simulink model "model"  (R2020b)
settings: Solver=VariableStepAuto  StartTime=0.0  StopTime=settings.Tsim  FixedStep=0.1  RelTol=1e-6  AbsTol=1e-6
values from neighbouring files (symbols this model uses):
  D = date(3)    [date2jd.m]
  settings = Simulink.Parameter    [main.m]
libraries: vrlib x10
(part 1 of 2)
settings Model: Creator=rosat  LastModifiedBy=rosat
settings SolverCC: ZeroCrossAlgorithm=Adaptive
settings OptimizationCC: BlockReduction=off  DefaultParameterBehavior=Inlined  BufferReuse=off
settings DebuggingCC: IgnoredZcDiagnostic=none  SFMachineParentedDataDiag=error

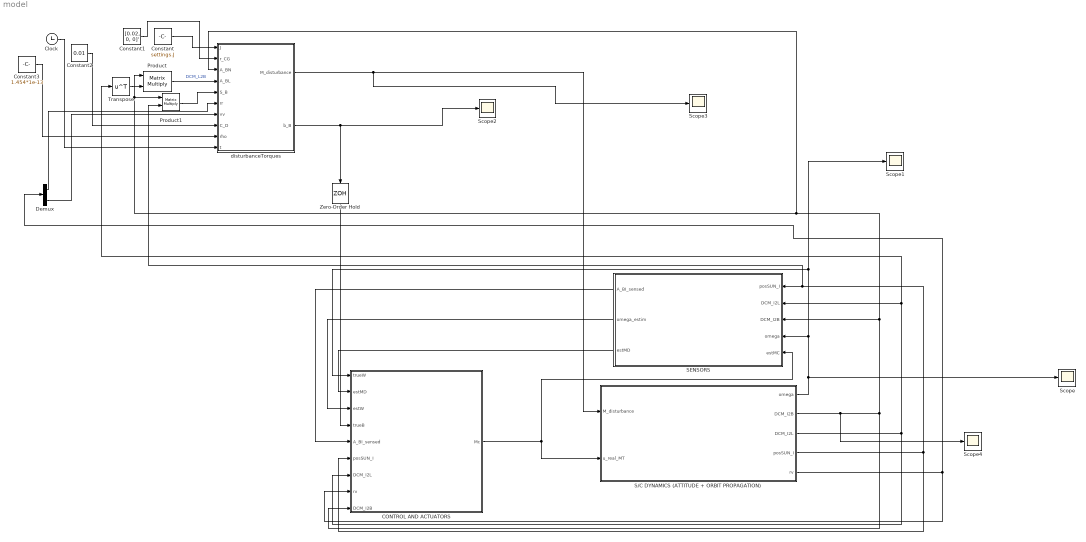
== system model ==
  CONTROL AND ACTUATORS : Subsystem
  Clock : Clock
  Constant : Constant  Value=settings.J
  Constant1 : Constant  Value=[0.02, 0, 0]'
  Constant2 : Constant  Value=0.01
  Constant3 : Constant  Value=1.454*1e-13
  Demux : Demux  Outputs=2
  Product : Product  Multiplication=Matrix(*)
  Product1 : Product  Multiplication=Matrix(*)
  S/C DYNAMICS (ATTITUDE + ORBIT PROPAGATION) : Subsystem
  SENSORS : Subsystem
  Scope{,1..4} (5 alike) : Scope
  Transpose : Math  Operator=transpose  SaturateOnIntegerOverflow=on
  Zero-Order Hold : ZeroOrderHold  SampleTime=0.01
  disturbanceTorques : MATLAB Function  TreatAsAtomicUnit=on
  wires:
  Constant/1 -> disturbanceTorques/1(J)
  Constant1/1 -> disturbanceTorques/2(r_CG)
  Transpose/1 -> Product/2
  Product/1 -> disturbanceTorques/4(A_BL)  "DCM_L2B"
  Product1/1 -> disturbanceTorques/5(S_B)
  Demux/1 -> disturbanceTorques/6(rr)
  Demux/2 -> disturbanceTorques/7(vv)
  Constant2/1 -> disturbanceTorques/8(C_D)
  Constant3/1 -> disturbanceTorques/9(rho)
  Clock/1 -> disturbanceTorques/10(t)
  disturbanceTorques/1(M_disturbance) -> Scope3/1, S/C DYNAMICS (ATTITUDE + ORBIT PROPAGATION)/1(M_disturbance)
  disturbanceTorques/2(b_B) -> Scope2/1, Zero-Order Hold/1
  Zero-Order Hold/1 -> CONTROL AND ACTUATORS/4(trueB)
  S/C DYNAMICS (ATTITUDE + ORBIT PROPAGATION)/3(DCM_I2L) -> Transpose/1, SENSORS/2(DCM_I2L), CONTROL AND ACTUATORS/7(DCM_I2L)
  S/C DYNAMICS (ATTITUDE + ORBIT PROPAGATION)/4(posSUN_I) -> Product1/2, SENSORS/1(posSUN_I), CONTROL AND ACTUATORS/6(posSUN_I)
  S/C DYNAMICS (ATTITUDE + ORBIT PROPAGATION)/1(omega) -> Scope1/1, CONTROL AND ACTUATORS/1(trueW), SENSORS/4(omega), Scope/1
  S/C DYNAMICS (ATTITUDE + ORBIT PROPAGATION)/2(DCM_I2B) -> Scope4/1, disturbanceTorques/3(A_BN), Product1/1, Product/1, SENSORS/3(DCM_I2B), CONTROL AND ACTUATORS/9(DCM_I2B)
  S/C DYNAMICS (ATTITUDE + ORBIT PROPAGATION)/5(rv) -> Demux/1, CONTROL AND ACTUATORS/8(rv)
  SENSORS/2(omega_estim) -> CONTROL AND ACTUATORS/3(estW)
  SENSORS/3(estMD) -> CONTROL AND ACTUATORS/2(estMD)
  SENSORS/1(A_BI_sensed) -> CONTROL AND ACTUATORS/5(A_BI_sensed)
  CONTROL AND ACTUATORS/1(Mc) -> S/C DYNAMICS (ATTITUDE + ORBIT PROPAGATION)/2(u_real_MT), SENSORS/5(estMC)

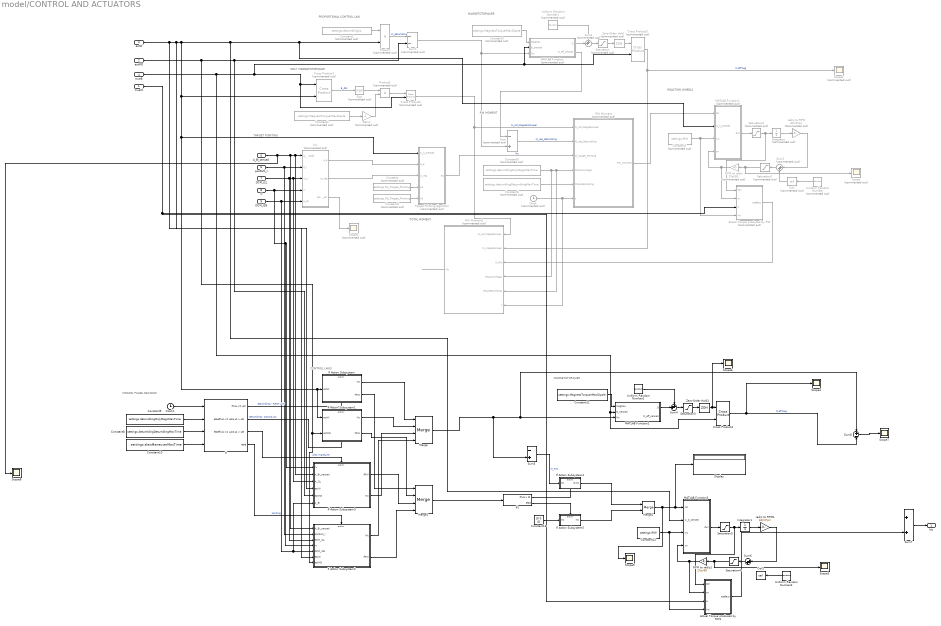
== system model/CONTROL AND ACTUATORS ==
  note: CONTROL LAWS
  note: MISSION PHASE DECISION
  note: TOTAL MOMENT
  note: REACTION WHEELS
  note: RW MOMENT
  note: TARGET POINTING
  note: MAGNETOTORQUER
  note: ONLY MAGNETOTORQUER
  note: PROPORTIONAL CONTROL LAW
  note: MAGNETOTORQUER
  trueW : Inport
  estMD : Inport  Port=2
  estW : Inport  Port=3
  trueB : Inport  Port=4
  A_BI_sensed : Inport  Port=5
  posSUN_I : Inport  Port=6
  DCM_I2L : Inport  Port=7
  rv : Inport  Port=8
  DCM_I2B : Inport  Port=9
  Actual Torque produced by RW : MATLAB Function  Commented=on  TreatAsAtomicUnit=on
  Actual Torque produced by RW1 : MATLAB Function  TreatAsAtomicUnit=on
  Ceil : Rounding  Commented=on  Operator=ceil
  Ceil1 : Rounding  Operator=ceil
  Clock : Clock  Commented=on
  Clock1 : Clock
  Constant : Constant  Commented=on  Value=settings.Kp_Target_Pointing
  Constant1 : Constant  Commented=on  Value=settings.detumblingkp
  Constant10 : Constant  Value=settings.slewManeuverMaxTime
  Constant11 : Constant  Value=settings.MagnetoTorquerMaxDipole
  Constant12 : Constant  Value=settings.IRW
  Constant13 : Constant  Value=[0 0 0]
  Constant2 : Constant  Commented=on  Value=settings.MagnetoTorquerMaxDipole
  Constant3 : Constant  Commented=on  Value=settings.MagnetoTorquerMaxDipole
  Constant4 : Constant  Commented=on  Value=settings.Kd_Target_Pointing
  Constant5 : Constant  Commented=on  Value=settings.detumblingOnlyMagnMaxTime
  Constant6 : Constant  Commented=on  Value=settings.detumblingDetumblingMaxTime
  Constant7 : Constant  Commented=on  Value=settings.IRW
  Constant8 : Constant  Value=settings.detumblingDetumblingMaxTime
  Constant9 : Constant  Value=settings.detumblingOnlyMagnMaxTime
  Cross Product1 : vrlib/Utilities/Cross Product  Commented=on
  Cross Product2 : vrlib/Utilities/Cross Product  Commented=on
  Cross Product3 : vrlib/Utilities/Cross Product  Commented=on
  Cross Product4 : vrlib/Utilities/Cross Product
  Display : Display
  Gain1 : Gain  Commented=on  Gain=-1
  If : If  NumInputs=4  IfExpression=u1 <= u2  ElseIfExpressions=u1 <= u3 & u1 > u2, u1 <= u4 & u1 > u3
  If Action Subsystem : Subsystem  TreatAsAtomicUnit=on
  If Action Subsystem1 : Subsystem  TreatAsAtomicUnit=on
  If Action Subsystem2 : Subsystem  TreatAsAtomicUnit=on
  If Action Subsystem3 : Subsystem  TreatAsAtomicUnit=on
  If Action Subsystem4 : Subsystem  TreatAsAtomicUnit=on
  If Action Subsystem5 : Subsystem  TreatAsAtomicUnit=on
  If1 : If
  Integrator : Integrator  Commented=on  InitialCondition=[0;0;0]
  Integrator1 : Integrator  InitialCondition=[0;0;0]
  MATLAB Function : MATLAB Function  Commented=on  TreatAsAtomicUnit=on
  MATLAB Function1 : MATLAB Function  Commented=on  TreatAsAtomicUnit=on
  MATLAB Function2 : MATLAB Function  TreatAsAtomicUnit=on
  MATLAB Function3 : MATLAB Function  TreatAsAtomicUnit=on
  Merge : Merge  Inputs=4
  Merge1 : Merge  Inputs=4
  Merge2 : Merge
  Product : Product  Commented=on
  Product1 : Product  Commented=on
  RPM to rad/s : Gain  Commented=on  Gain=2*pi/60
  RPM to rad/s1 : Gain  Gain=2*pi/60
  RW Moment : MATLAB Function  Commented=on  TreatAsAtomicUnit=on
  RW Moment1 : MATLAB Function  Commented=on  TreatAsAtomicUnit=on
  Saturation : Saturate  Commented=on  UpperLimit=settings.MagnetoTorquerMaxDipole  LowerLimit=-settings.MagnetoTorquerMaxDipole
  Saturation1 : Saturate  Commented=on  UpperLimit=settings.MaxRPM*[1;1;1]  LowerLimit=-settings.MaxRPM*[1;1;1]  LinearizeAsGain=off  ZeroCross=off
  Saturation2 : Saturate  Commented=on  UpperLimit=settings.MaxRPM_Rate  LowerLimit=-settings.MaxRPM_Rate
  Saturation3 : Saturate  UpperLimit=settings.MagnetoTorquerMaxDipole  LowerLimit=-settings.MagnetoTorquerMaxDipole
  Saturation4 : Saturate  UpperLimit=settings.MaxRPM*[1;1;1]  LowerLimit=-settings.MaxRPM*[1;1;1]  LinearizeAsGain=off  ZeroCross=off
  Saturation5 : Saturate  UpperLimit=settings.MaxRPM_Rate  LowerLimit=-settings.MaxRPM_Rate
  Scope : Scope  Commented=on
  Scope1 : Scope  Commented=on
  Scope2 : Scope  Commented=on
  Scope{3..8} (6 alike) : Scope
  Sign : Signum  Commented=on
  Sum : Sum  Commented=on  Inputs=-+
  Sum1 : Sum  Commented=on  Inputs=--
  Sum2 : Sum  Commented=on  Inputs=++|
  Sum3 : Sum  Commented=on  Inputs=|++
  Sum4 : Sum  Inputs=++|
  Sum5 : Sum  Inputs=-+
  Sum6 : Sum  Inputs=|++
  Sum7 : Sum
  Sum8 : Sum  Inputs=+-
  Target Pointing Algorithm : MATLAB Function  Commented=on  TreatAsAtomicUnit=on
  Uniform Random Number : UniformRandomNumber  Commented=on  Minimum=-settings.RPMAccuracy*[1;1;1]  Maximum=settings.RPMAccuracy*[1;1;1]  Seed=561651  SampleTime=1/settings.RW_sr
  Uniform Random Number1 : UniformRandomNumber  Commented=on  Minimum=-settings.MagnetoTorquerDipoleError*[1;1;1]  Maximum=settings.MagnetoTorquerDipoleError*[1;1;1]  Seed=456156  SampleTime=1/settings.MagnetoTorquerSampleRate
  Uniform Random Number2 : UniformRandomNumber  Minimum=-settings.MagnetoTorquerDipoleError*[1;1;1]  Maximum=settings.MagnetoTorquerDipoleError*[1;1;1]  Seed=456156  SampleTime=1/settings.MagnetoTorquerSampleRate
  Uniform Random Number3 : UniformRandomNumber  Minimum=-settings.RPMAccuracy*[1;1;1]  Maximum=settings.RPMAccuracy*[1;1;1]  Seed=561651  SampleTime=1/settings.RW_sr
  Zero-Order Hold : ZeroOrderHold  Commented=on  SampleTime=1/settings.MagnetoTorquerSampleRate
  Zero-Order Hold1 : ZeroOrderHold  SampleTime=1/settings.MagnetoTorquerSampleRate
  fcn : MATLAB Function  Commented=on  TreatAsAtomicUnit=on
  rad/s to RPM : Gain  Commented=on  Gain=60/(2*pi)
  rad/s to RPM1 : Gain  Gain=60/(2*pi)
  Mc : Outport
  wires:
  Constant1/1 -> Product/1
  Cross Product2/1 -> RW Moment1/1(M_onlyMagnetorquer), RW Moment/1(M_onlyMagnetorquer)  "M_onlyMagnetotorquer"
  Constant2/1 -> Gain1/1
  Cross Product1/1 -> Sign/1  "B_dot"
  Gain1/1 -> Product1/2
  Sign/1 -> Product1/1
  Product1/1 -> Cross Product2/1
  MATLAB Function/2(M_eff_sensed) -> Sum/1
  Uniform Random Number1/1 -> Sum2/1
  Zero-Order Hold/1 -> Cross Product3/1
  MATLAB Function/1(D) -> Sum2/2
  Sum2/1 -> Saturation/1
  Saturation/1 -> Zero-Order Hold/1
  Cross Product3/1 -> Scope1/1, RW Moment1/2(M_magnetorquer)  "M eff Mag"
  Constant3/1 -> MATLAB Function/1(MagMax)
  Sum/1 -> RW Moment/2(M_req_Detumbling)  "M_req_detumbling"
  Product/1 -> Sum1/1  "M_detumbling"
  Sum1/1 -> Sum/2, MATLAB Function/3(Mc)
  fcn/1(A_e) -> Target Pointing Algorithm/2(A_e)
  DCM_I2L/1 -> If Action Subsystem2/3(DCM_I2L), If Action Subsystem3/3(A_I2L), fcn/3(A_LI)
  Target Pointing Algorithm/1(Mc) -> RW Moment/3(M_Target_Pointing)  "Mc"
  A_BI_sensed/1 -> Scope8/1, If Action Subsystem3/2(A_BI_sensed), fcn/1(A_BI_sensed), If Action Subsystem2/1(A_BI_sensed)
  Constant/1 -> Target Pointing Algorithm/4(Kp)
  Constant4/1 -> Target Pointing Algorithm/5(Kd)
  posSUN_I/1 -> If Action Subsystem2/2(posSUN_I), fcn/2(S_I)
  DCM_I2B/1 -> If Action Subsystem3/6(A_BI), If Action Subsystem2/5(DCM_I2B), fcn/5(A_BI)
  fcn/3(pointing_err) -> Scope2/1
  rv/1 -> If Action Subsystem3/1(rv), If Action Subsystem2/4(rv), fcn/4(rv)
  fcn/2(w_req) -> Target Pointing Algorithm/3(w_req)
  Constant5/1 -> RW Moment1/4(tMaxOnlyMagn), RW Moment1/5(tMaxDetumbling), RW Moment/4(tMaxOnlyMagn)
  Constant6/1 -> RW Moment/5(tMaxDetumbling)
  Clock/1 -> RW Moment1/6(t), RW Moment/6(t)
  RW Moment/1(RW_Moment) -> MATLAB Function1/1(Mc)
  Actual Torque produced by RW/1(MeffRW) -> RW Moment1/3(M_RW)
  Ceil/1 -> Sum3/2
  Sum3/1 -> Saturation1/1
  Saturation1/1 -> Scope/1, RPM to rad/s/1
  Integrator/1 -> rad/s to RPM/1
  MATLAB Function1/1(dwr) -> Saturation2/1
  Constant7/1 -> Actual Torque produced by RW/4(Irw), MATLAB Function1/3(Irw)
  RPM to rad/s/1 -> Actual Torque produced by RW/2(wr), MATLAB Function1/4(wr)
  trueW/1 -> Actual Torque produced by RW1/3(w), Actual Torque produced by RW/3(w)
  Uniform Random Number/1 -> Ceil/1
  rad/s to RPM/1 -> Sum3/1
  Saturation2/1 -> Actual Torque produced by RW/1(dwr), Integrator/1
  RW Moment1/1(Mc) -> ?
  Clock1/1 -> If/1
  Constant9/1 -> If/2
  Constant8/1 -> If/3
  If/1 -> If Action Subsystem/Action  "detumbling - FIRST LAW"
  If/2 -> If Action Subsystem1/Action  "detumbling - second law"
  If/4 -> If Action Subsystem2/Action  "pointing"
  Constant10/1 -> If/4
  If/3 -> If Action Subsystem3/Action  "slew maneuver"
  estW/1 -> If Action Subsystem2/6(estW), If Action Subsystem3/4(estW), If Action Subsystem1/1(estW), If Action Subsystem/1(estW), Target Pointing Algorithm/1(w_b_sensed), Cross Product1/2, MATLAB Function3/2(w_b_sensed), MATLAB Function1/2(w_b_sensed), Product/2
  trueB/1 -> Cross Product4/2, MATLAB Function2/2(B_sensed), Cross Product3/2, MATLAB Function/2(B_sensed), Cross Product2/2, Cross Product1/1
  Sum4/1 -> Saturation3/1
  Zero-Order Hold1/1 -> Scope6/1, Cross Product4/1
  Constant11/1 -> MATLAB Function2/1(MagMax)
  MATLAB Function2/1(D) -> Sum4/2
  Saturation3/1 -> Zero-Order Hold1/1
  Uniform Random Number2/1 -> Sum4/1
  If Action Subsystem/1(Mc) -> Merge/1
  If Action Subsystem1/1(Mc) -> Merge/2
  If Action Subsystem/2(ifRW) -> Merge1/1
  If Action Subsystem1/2(ifRW) -> Merge1/2
  If Action Subsystem2/2(ifRW) -> Merge1/4
  If Action Subsystem2/1(Mc) -> Merge/4
  If Action Subsystem3/2(Mc) -> Merge/3
  If Action Subsystem3/1(ifRW) -> Merge1/3
  Merge/1 -> Sum5/2, Sum8/1, MATLAB Function2/3(Mc)
  estMD/1 -> If Action Subsystem2/7(estMD), If Action Subsystem1/2(estMD), If Action Subsystem3/5(estMD), Sum1/2
  Merge1/1 -> If1/1
  Cross Product4/1 -> Scope4/1, Sum8/2  "M eff Mag"
  Sum5/1 -> If Action Subsystem4/1(In1)  "M_RW"
  rad/s to RPM1/1 -> Sum6/1
  Uniform Random Number3/1 -> Ceil1/1
  RPM to rad/s1/1 -> Actual Torque produced by RW1/2(wr), MATLAB Function3/4(wr)
  Constant12/1 -> Actual Torque produced by RW1/4(Irw), MATLAB Function3/3(Irw)
  MATLAB Function3/1(dwr) -> Saturation5/1
  Saturation4/1 -> Scope3/1, RPM to rad/s1/1
  Sum6/1 -> Saturation4/1
  Integrator1/1 -> rad/s to RPM1/1
  Saturation5/1 -> Actual Torque produced by RW1/1(dwr), Integrator1/1
  If1/1 -> If Action Subsystem4/Action
  If1/2 -> If Action Subsystem5/Action
  Constant13/1 -> If Action Subsystem5/1(In1)
  Merge2/1 -> Scope5/1, Display/1, MATLAB Function3/1(Mc)
  If Action Subsystem4/1(Out1) -> Merge2/1
  If Action Subsystem5/1(Mc) -> Merge2/2
  Sum7/1 -> Mc/1
  Sum8/1 -> Scope7/1
  Actual Torque produced by RW1/1(MeffRW) -> Sum7/2

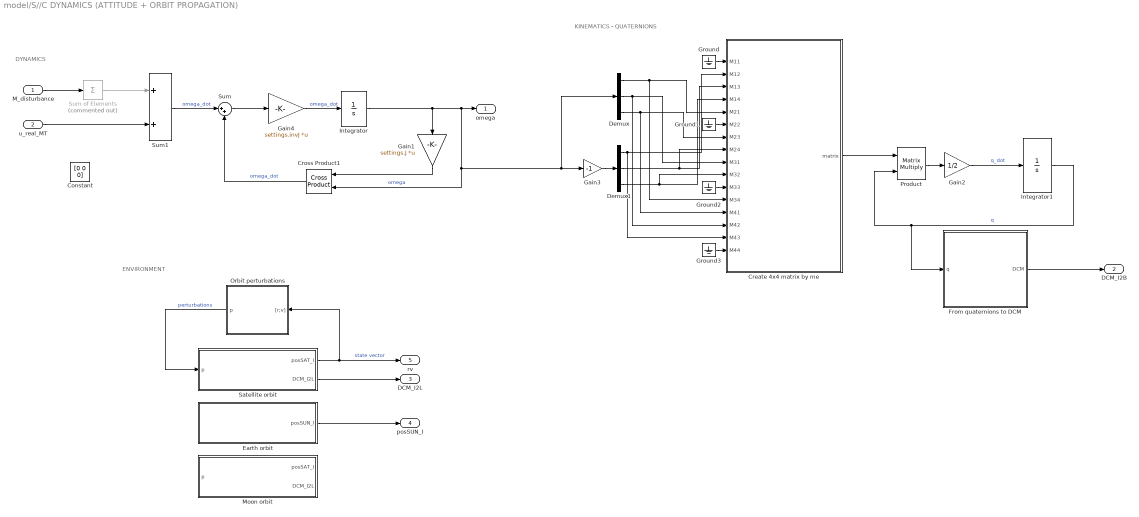
== system model/S//C DYNAMICS (ATTITUDE + ORBIT PROPAGATION) ==
  note: ENVIRONMENT
  note: KINEMATICS - QUATERNIONS
  note: DYNAMICS
  M_disturbance : Inport
  u_real_MT : Inport  Port=2
  Constant : Constant  Value=[0 0 0]
  Create 4x4 matrix by me : Subsystem
  Cross Product1 : vrlib/Utilities/Cross Product
  Demux : Demux  Outputs=3
  Demux1 : Demux  Outputs=3
  Earth orbit : Subsystem
  From quaternions to DCM : Subsystem
  Gain1 : Gain  Gain=settings.J  Multiplication=Matrix(K*u)
  Gain2 : Gain  Gain=1/2
  Gain3 : Gain  Gain=-1
  Gain4 : Gain  Gain=settings.invJ  Multiplication=Matrix(K*u)
  Ground{,1..3} (4 alike) : Ground
  Integrator : Integrator  InitialCondition=settings.omega0
  Integrator1 : Integrator  InitialCondition=settings.q0
  Moon orbit : Subsystem
  Orbit perturbations : Subsystem
  Product : Product  Multiplication=Matrix(*)
  Satellite orbit : Subsystem
  Sum : Sum  Inputs=|++
  Sum of Elements : Sum  Commented=on  Inputs=+  CollapseMode=Specified dimension  CollapseDim=2
  Sum1 : Sum
  omega : Outport
  DCM_I2B : Outport  Port=2
  DCM_I2L : Outport  Port=3
  posSUN_I : Outport  Port=4
  rv : Outport  Port=5
  wires:
  Sum of Elements/1 -> Sum1/1
  Integrator/1 -> Gain1/1, Demux/1, Gain3/1, Cross Product1/2, omega/1  "omega"
  Sum/1 -> Gain4/1
  u_real_MT/1 -> Sum1/2
  Sum1/1 -> Sum/1  "omega_dot"
  Gain4/1 -> Integrator/1  "omega_dot"
  Cross Product1/1 -> Sum/2  "omega_dot"
  Gain1/1 -> Cross Product1/1
  M_disturbance/1 -> Sum of Elements/1
  Demux/3 -> Create 4x4 matrix by me/13(M41), Create 4x4 matrix by me/7(M23)
  Product/1 -> Gain2/1
  Demux1/2 -> Create 4x4 matrix by me/8(M24), Create 4x4 matrix by me/3(M13)
  Demux1/3 -> Create 4x4 matrix by me/10(M32), Create 4x4 matrix by me/4(M14)
  Demux1/1 -> Create 4x4 matrix by me/15(M43), Create 4x4 matrix by me/2(M12)
  Demux/1 -> Create 4x4 matrix by me/12(M34), Create 4x4 matrix by me/5(M21)
  Ground2/1 -> Create 4x4 matrix by me/11(M33)
  Ground/1 -> Create 4x4 matrix by me/1(M11)
  From quaternions to DCM/1(DCM) -> DCM_I2B/1
  Demux/2 -> Create 4x4 matrix by me/14(M42), Create 4x4 matrix by me/9(M31)
  Ground3/1 -> Create 4x4 matrix by me/16(M44)
  Gain2/1 -> Integrator1/1  "q_dot"
  Integrator1/1 -> From quaternions to DCM/1(q), Product/2  "q"
  Gain3/1 -> Demux1/1
  Ground1/1 -> Create 4x4 matrix by me/6(M22)
  Create 4x4 matrix by me/1(matrix) -> Product/1
  Earth orbit/1(posSUN_I) -> posSUN_I/1
  Satellite orbit/1(posSAT_I) -> Orbit perturbations/1("[r;v]"), rv/1  "state vector"
  Orbit perturbations/1(p) -> Satellite orbit/1(p)  "perturbations"
  Satellite orbit/2(DCM_I2L) -> DCM_I2L/1

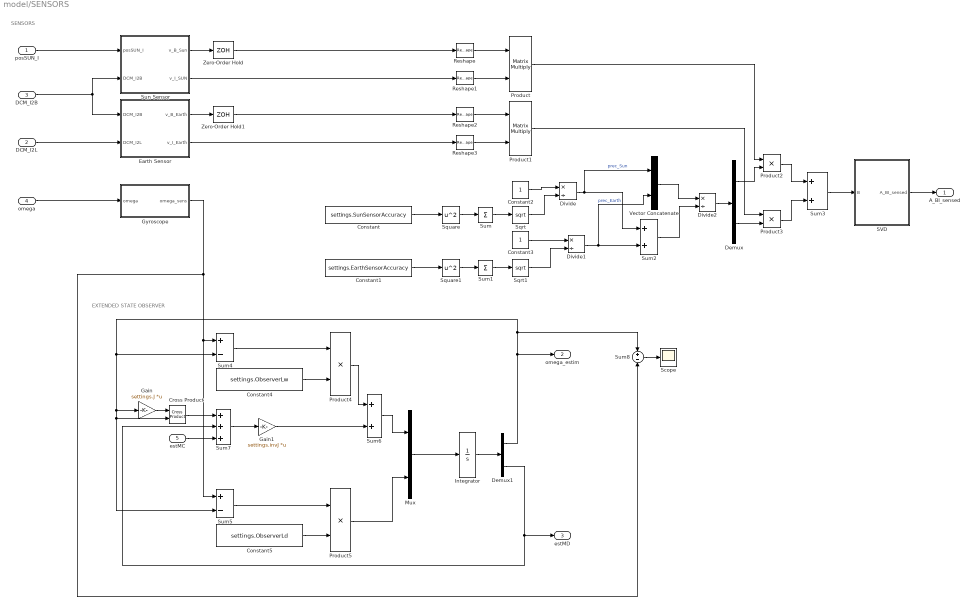
== system model/SENSORS ==
  note: EXTENDED STATE OBSERVER
  note: SENSORS
  posSUN_I : Inport
  DCM_I2L : Inport  Port=2
  DCM_I2B : Inport  Port=3
  omega : Inport  Port=4
  estMC : Inport  Port=5
  Constant : Constant  Value=settings.SunSensorAccuracy
  Constant1 : Constant  Value=settings.EarthSensorAccuracy
  Constant2 : Constant
  Constant3 : Constant
  Constant4 : Constant  Value=settings.ObserverLw
  Constant5 : Constant  Value=settings.ObserverLd
  Cross Product : vrlib/Utilities/Cross Product
  Demux : Demux  Outputs=2
  Demux1 : Demux  Outputs=2
  Divide : Product  Inputs=*/
  Divide1 : Product  Inputs=*/
  Divide2 : Product  Inputs=*/
  Earth Sensor : Subsystem
  Gain : Gain  Gain=settings.J  Multiplication=Matrix(K*u)
  Gain1 : Gain  Gain=settings.invJ  Multiplication=Matrix(K*u)
  Gyroscope : Subsystem
  Integrator : Integrator  InitialCondition=[settings.omega0; settings.ObserverMd0]
  Mux : Mux  Inputs=2
  Product : Product  Multiplication=Matrix(*)
  Product1 : Product  Multiplication=Matrix(*)
  Product{2..5} (4 alike) : Product
  Reshape : Reshape  OutputDimensionality=Column vector (2-D)
  Reshape1 : Reshape  OutputDimensionality=Row vector (2-D)
  Reshape2 : Reshape  OutputDimensionality=Column vector (2-D)
  Reshape3 : Reshape  OutputDimensionality=Row vector (2-D)
  SVD : MATLAB Function  TreatAsAtomicUnit=on
  Scope : Scope
  Sqrt : Sqrt  SaturateOnIntegerOverflow=on
  Sqrt1 : Sqrt  SaturateOnIntegerOverflow=on
  Square : Math  Operator=square  SaturateOnIntegerOverflow=on
  Square1 : Math  Operator=square  SaturateOnIntegerOverflow=on
  Sum : Sum  Inputs=+
  Sum1 : Sum  Inputs=+
  Sum2 : Sum
  Sum3 : Sum
  Sum4 : Sum  Inputs=+-
  Sum5 : Sum  Inputs=+-
  Sum6 : Sum
  Sum7 : Sum  Inputs=+++
  Sum8 : Sum  Inputs=+-
  Sun Sensor : Subsystem
  Vector Concatenate : Concatenate
  Zero-Order Hold : ZeroOrderHold  SampleTime=1/settings.SunSensorSampleRate
  Zero-Order Hold1 : ZeroOrderHold  SampleTime=1/settings.EarthSensorSampleRate
  A_BI_sensed : Outport
  omega_estim : Outport  Port=2
  estMD : Outport  Port=3
  wires:
  DCM_I2B/1 -> Sun Sensor/2(DCM_I2B), Earth Sensor/1(DCM_I2B)
  posSUN_I/1 -> Sun Sensor/1(posSUN_I)
  DCM_I2L/1 -> Earth Sensor/2(DCM_I2L)
  Sun Sensor/1(v_B_Sun) -> Zero-Order Hold/1
  Earth Sensor/1(v_B_Earth) -> Zero-Order Hold1/1
  omega/1 -> Gyroscope/1(omega)
  Gyroscope/1(omega_sens) -> Sum8/2, Sum5/1, Sum4/1
  Product3/1 -> Sum3/2
  Sum3/1 -> SVD/1(B)
  Demux/1 -> Product2/2
  Product2/1 -> Sum3/1
  Sum/1 -> Sqrt/1
  Square/1 -> Sum/1
  Sum2/1 -> Divide2/2
  Reshape2/1 -> Product1/1
  Constant1/1 -> Square1/1
  Sqrt/1 -> Divide/2
  Sun Sensor/2(v_I_SUN) -> Reshape1/1
  Sum1/1 -> Sqrt1/1
  Reshape3/1 -> Product1/2
  Product1/1 -> Product3/1
  Earth Sensor/2(v_I_Earth) -> Reshape3/1
  Reshape/1 -> Product/1
  Zero-Order Hold/1 -> Reshape/1
  Divide1/1 -> Sum2/2, Vector Concatenate/2  "prec_Earth"
  Zero-Order Hold1/1 -> Reshape2/1
  Divide2/1 -> Demux/1
  Sqrt1/1 -> Divide1/2
  Demux/2 -> Product3/2
  Reshape1/1 -> Product/2
  Constant/1 -> Square/1
  Divide/1 -> Sum2/1, Vector Concatenate/1  "prec_Sun"
  Square1/1 -> Sum1/1
  Product/1 -> Product2/1
  SVD/1(A_BI_sensed) -> A_BI_sensed/1
  Vector Concatenate/1 -> Divide2/1
  Constant2/1 -> Divide/1
  Constant3/1 -> Divide1/1
  Sum4/1 -> Product4/1
  Constant4/1 -> Product4/2
  Constant5/1 -> Product5/2
  Sum5/1 -> Product5/1
  Integrator/1 -> Demux1/1
  Demux1/1 -> omega_estim/1, Sum8/1, Sum5/2, Cross Product/2, Gain/1, Sum4/2
  Product4/1 -> Sum6/1
  Gain/1 -> Cross Product/1
  Cross Product/1 -> Sum7/1
  Demux1/2 -> estMD/1, Sum7/2
  Sum7/1 -> Gain1/1
  Gain1/1 -> Sum6/2
  Sum6/1 -> Mux/1
  Product5/1 -> Mux/2
  Mux/1 -> Integrator/1
  estMC/1 -> Sum7/3
  Sum8/1 -> Scope/1

== system model/CONTROL AND ACTUATORS/If Action Subsystem ==
  estW : Inport
  Action Port : ActionPort  ActionPortLabel=if(u1 <= u2)
  Constant : Constant  Value=settings.detumblingkb
  Constant1 : Constant  Value=0
  Gain : Gain  Gain=-1
  Product : Product
  Mc : Outport
  ifRW : Outport  Port=2
  wires:
  estW/1 -> Product/1
  Constant/1 -> Product/2
  Product/1 -> Gain/1
  Constant1/1 -> ifRW/1
  Gain/1 -> Mc/1

== system model/CONTROL AND ACTUATORS/If Action Subsystem1 ==
  estW : Inport
  estMD : Inport  Port=2
  Action Port : ActionPort  ActionPortLabel=elseif(u1 <= u3 & u1 > u2)
  Constant : Constant  Value=settings.detumblingkp
  Constant1 : Constant
  Product : Product
  Sum : Sum  Inputs=--
  Mc : Outport
  ifRW : Outport  Port=2
  wires:
  estW/1 -> Product/1
  Constant/1 -> Product/2
  Product/1 -> Sum/1
  estMD/1 -> Sum/2
  Sum/1 -> Mc/1
  Constant1/1 -> ifRW/1

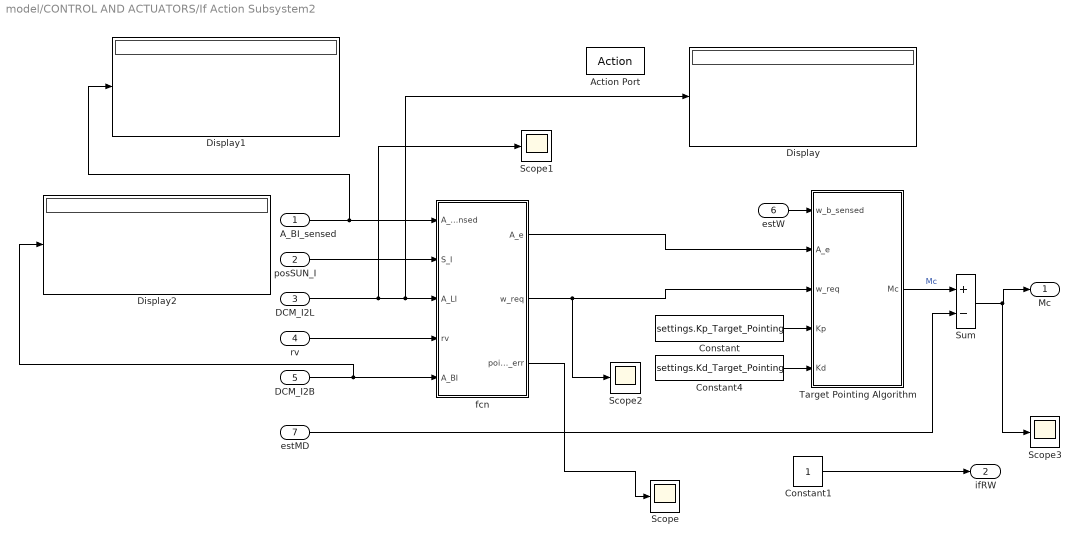
== system model/CONTROL AND ACTUATORS/If Action Subsystem2 ==
  A_BI_sensed : Inport
  posSUN_I : Inport  Port=2
  DCM_I2L : Inport  Port=3
  rv : Inport  Port=4
  DCM_I2B : Inport  Port=5
  estW : Inport  Port=6
  estMD : Inport  Port=7
  Action Port : ActionPort  ActionPortLabel=else
  Constant : Constant  Value=settings.Kp_Target_Pointing
  Constant1 : Constant
  Constant4 : Constant  Value=settings.Kd_Target_Pointing
  Display : Display
  Display1 : Display
  Display2 : Display
  Scope{,1..3} (4 alike) : Scope
  Sum : Sum  Inputs=+-
  Target Pointing Algorithm : MATLAB Function  TreatAsAtomicUnit=on
  fcn : MATLAB Function  TreatAsAtomicUnit=on
  Mc : Outport
  ifRW : Outport  Port=2
  wires:
  fcn/3(pointing_err) -> Scope/1
  fcn/1(A_e) -> Target Pointing Algorithm/2(A_e)
  estW/1 -> Target Pointing Algorithm/1(w_b_sensed)
  Constant4/1 -> Target Pointing Algorithm/5(Kd)
  fcn/2(w_req) -> Scope2/1, Target Pointing Algorithm/3(w_req)
  posSUN_I/1 -> fcn/2(S_I)
  rv/1 -> fcn/4(rv)
  Constant/1 -> Target Pointing Algorithm/4(Kp)
  Constant1/1 -> ifRW/1
  Target Pointing Algorithm/1(Mc) -> Sum/1  "Mc"
  estMD/1 -> Sum/2
  Sum/1 -> Scope3/1, Mc/1
  DCM_I2L/1 -> Scope1/1, Display/1, fcn/3(A_LI)
  A_BI_sensed/1 -> fcn/1(A_BI_sensed), Display1/1
  DCM_I2B/1 -> Display2/1, fcn/5(A_BI)

== system model/CONTROL AND ACTUATORS/If Action Subsystem3 ==
  rv : Inport
  A_BI_sensed : Inport  Port=2
  A_I2L : Inport  Port=3
  estW : Inport  Port=4
  estMD : Inport  Port=5
  A_BI : Inport  Port=6
  Action Port : ActionPort  ActionPortLabel=elseif( u1 <= u4 & u1 > u3)
  Constant : Constant  Value=settings.slewMank1
  Constant1 : Constant
  Constant2 : Constant  Value=settings.slewMank2
  Constant3 : Constant  Value=settings.J
  MATLAB Function : MATLAB Function  TreatAsAtomicUnit=on
  MATLAB Function1 : MATLAB Function  TreatAsAtomicUnit=on
  Scope : Scope
  ifRW : Outport
  Mc : Outport  Port=2
  wires:
  Constant1/1 -> ifRW/1
  rv/1 -> MATLAB Function/1(rv)
  estW/1 -> MATLAB Function1/3(estW), MATLAB Function/4(estW)
  A_I2L/1 -> MATLAB Function/3(A_LI)
  A_BI_sensed/1 -> MATLAB Function/2(A_BI_sensed)
  estMD/1 -> MATLAB Function1/4(estMD)
  MATLAB Function/1(w_e) -> MATLAB Function1/1(w_e)
  MATLAB Function/2(A_e) -> MATLAB Function1/2(A_e)
  MATLAB Function1/1(Mc) -> Mc/1
  Constant/1 -> MATLAB Function1/5(k1)
  Constant2/1 -> MATLAB Function1/6(k2)
  Constant3/1 -> MATLAB Function1/7(J)
  A_BI/1 -> MATLAB Function/5(A_BI)
  MATLAB Function/3(pointing_err) -> Scope/1

== system model/CONTROL AND ACTUATORS/If Action Subsystem4 ==
  In1 : Inport
  Action Port : ActionPort  ActionPortLabel=if(u1 > 0)
  Out1 : Outport
  wires:
  In1/1 -> Out1/1

== system model/CONTROL AND ACTUATORS/If Action Subsystem5 ==
  In1 : Inport
  Action Port : ActionPort  ActionPortLabel=else
  Mc : Outport
  wires:
  In1/1 -> Mc/1

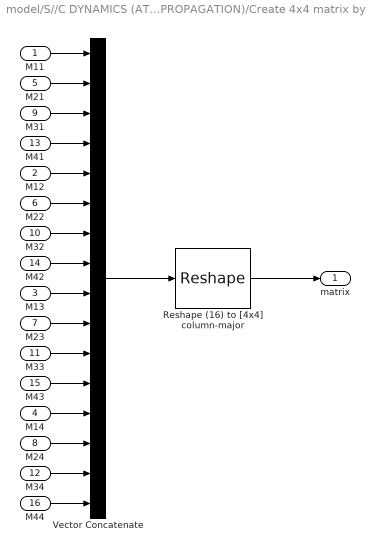
== system model/S//C DYNAMICS (ATTITUDE + ORBIT PROPAGATION)/Create 4x4 matrix by me ==
  M11 : Inport
  M12 : Inport  Port=2
  M13 : Inport  Port=3
  M14 : Inport  Port=4
  M21 : Inport  Port=5
  M22 : Inport  Port=6
  M23 : Inport  Port=7
  M24 : Inport  Port=8
  M31 : Inport  Port=9
  M32 : Inport  Port=10
  M33 : Inport  Port=11
  M34 : Inport  Port=12
  M41 : Inport  Port=13
  M42 : Inport  Port=14
  M43 : Inport  Port=15
  M44 : Inport  Port=16
  Reshape (16) to [4x4] column-major : Reshape  OutputDimensionality=Customize  OutputDimensions=[4,4]
  Vector Concatenate : Concatenate  NumInputs=16
  matrix : Outport
  wires:
  M12/1 -> Vector Concatenate/5
  M11/1 -> Vector Concatenate/1
  M13/1 -> Vector Concatenate/9
  M14/1 -> Vector Concatenate/13
  M21/1 -> Vector Concatenate/2
  M44/1 -> Vector Concatenate/16
  M34/1 -> Vector Concatenate/15
  M24/1 -> Vector Concatenate/14
  M43/1 -> Vector Concatenate/12
  M33/1 -> Vector Concatenate/11
  M23/1 -> Vector Concatenate/10
  M42/1 -> Vector Concatenate/8
  M32/1 -> Vector Concatenate/7
  M22/1 -> Vector Concatenate/6
  M41/1 -> Vector Concatenate/4
  M31/1 -> Vector Concatenate/3
  Vector Concatenate/1 -> Reshape (16) to [4x4] column-major/1
  Reshape (16) to [4x4] column-major/1 -> matrix/1

== system model/S//C DYNAMICS (ATTITUDE + ORBIT PROPAGATION)/Earth orbit ==
  Constant2 : Constant  Value=-settings.muS
  Constant3 : Constant  Value=3
  Demux : Demux  Outputs=2
  Demux1 : Demux  Outputs=2
  Divide1 : Product  Inputs=*/
  Gain : Gain  Gain=-1
  Integrator : Integrator  InitialCondition=settings.Y0E
  Mux : Mux  Inputs=2
  Product : Product
  Product1 : Product  Multiplication=Matrix(*)
  R_E2CI : Constant  Value=[1 0 0; 0 cosd(23.4) -sind(23.4); 0 sind(23.4) cosd(23.4)]  VectorParams1D=off
  Sqrt : Sqrt  SaturateOnIntegerOverflow=on
  Square : Math  Operator=square  SaturateOnIntegerOverflow=on
  Square1 : Math  Operator=pow  SaturateOnIntegerOverflow=on
  Sum : Sum  Inputs=+
  Terminator : Terminator
  posSUN_I : Outport
  wires:
  Constant3/1 -> Square1/2
  Demux/1 -> Product/1, Square/1  "r"
  Demux/2 -> Mux/1
  Integrator/1 -> Demux1/1, Demux/1  "[r;v]"
  Divide1/1 -> Product/2
  Sqrt/1 -> Square1/1  "r_norm"
  Constant2/1 -> Divide1/1
  Product/1 -> Mux/2
  Sum/1 -> Sqrt/1
  Square/1 -> Sum/1
  Square1/1 -> Divide1/2  "r_norm^3"
  Mux/1 -> Integrator/1  "[r_dot; v_dot]"
  Gain/1 -> Product1/2
  R_E2CI/1 -> Product1/1
  Demux1/1 -> Gain/1
  Demux1/2 -> Terminator/1
  Product1/1 -> posSUN_I/1

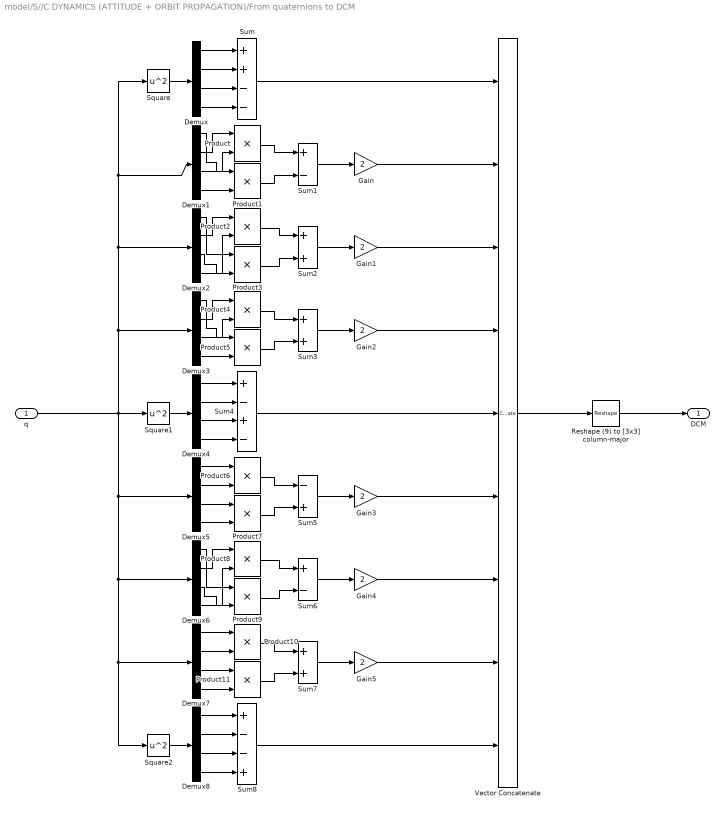
== system model/S//C DYNAMICS (ATTITUDE + ORBIT PROPAGATION)/From quaternions to DCM ==
  q : Inport
  Demux{,1..8} (9 alike) : Demux
  Gain{,1..5} (6 alike) : Gain  Gain=2
  Product{,1..11} (12 alike) : Product
  Reshape (9) to [3x3] column-major : Reshape  OutputDimensionality=Customize  OutputDimensions=[3,3]
  Square : Math  Operator=square  SaturateOnIntegerOverflow=on
  Square1 : Math  Operator=square  SaturateOnIntegerOverflow=on
  Square2 : Math  Operator=square  SaturateOnIntegerOverflow=on
  Sum : Sum  Inputs=++--
  Sum1 : Sum  Inputs=+-
  Sum2 : Sum
  Sum3 : Sum
  Sum4 : Sum  Inputs=+-+-
  Sum5 : Sum  Inputs=-+
  Sum6 : Sum  Inputs=+-
  Sum7 : Sum
  Sum8 : Sum  Inputs=+--+
  Vector Concatenate : Concatenate  NumInputs=9
  DCM : Outport
  wires:
  q/1 -> Square/1, Demux1/1, Demux2/1, Demux3/1, Square1/1, Demux5/1, Demux6/1, Demux7/1, Square2/1
  Vector Concatenate/1 -> Reshape (9) to [3x3] column-major/1
  Square/1 -> Demux/1
  Demux/3 -> Sum/3
  Demux/4 -> Sum/4
  Demux/2 -> Sum/2
  Demux/1 -> Sum/1
  Sum/1 -> Vector Concatenate/1
  Demux1/2 -> Product/1
  Demux1/3 -> Product/2
  Demux1/1 -> Product1/1
  Demux1/4 -> Product1/2
  Product/1 -> Sum1/1
  Product1/1 -> Sum1/2
  Sum1/1 -> Gain/1
  Gain/1 -> Vector Concatenate/2
  Demux2/2 -> Product2/1
  Demux2/4 -> Product2/2
  Demux2/1 -> Product3/1
  Demux2/3 -> Product3/2
  Product3/1 -> Sum2/2
  Product2/1 -> Sum2/1
  Sum2/1 -> Gain1/1
  Gain1/1 -> Vector Concatenate/3
  Demux3/1 -> Product5/1
  Product5/1 -> Sum3/2
  Demux3/2 -> Product4/1
  Product4/1 -> Sum3/1
  Demux3/3 -> Product4/2
  Demux3/4 -> Product5/2
  Sum3/1 -> Gain2/1
  Gain2/1 -> Vector Concatenate/4
  Demux4/3 -> Sum4/3
  Demux4/1 -> Sum4/1
  Demux4/4 -> Sum4/4
  Sum4/1 -> Vector Concatenate/5
  Demux4/2 -> Sum4/2
  Square1/1 -> Demux4/1
  Product7/1 -> Sum5/2
  Product6/1 -> Sum5/1
  Sum5/1 -> Gain3/1
  Demux5/3 -> Product7/1
  Demux5/4 -> Product7/2
  Demux5/1 -> Product6/1
  Demux5/2 -> Product6/2
  Gain3/1 -> Vector Concatenate/6
  Sum6/1 -> Gain4/1
  Demux6/2 -> Product8/1
  Gain4/1 -> Vector Concatenate/7
  Demux6/4 -> Product8/2
  Demux6/3 -> Product9/2
  Demux6/1 -> Product9/1
  Product9/1 -> Sum6/2
  Product8/1 -> Sum6/1
  Demux7/2 -> Product10/2
  Demux7/3 -> Product11/1
  Sum7/1 -> Gain5/1
  Product10/1 -> Sum7/1
  Demux7/1 -> Product10/1
  Demux7/4 -> Product11/2
  Product11/1 -> Sum7/2
  Gain5/1 -> Vector Concatenate/8
  Demux8/2 -> Sum8/2
  Square2/1 -> Demux8/1
  Sum8/1 -> Vector Concatenate/9
  Demux8/3 -> Sum8/3
  Reshape (9) to [3x3] column-major/1 -> DCM/1
  Demux8/1 -> Sum8/1
  Demux8/4 -> Sum8/4

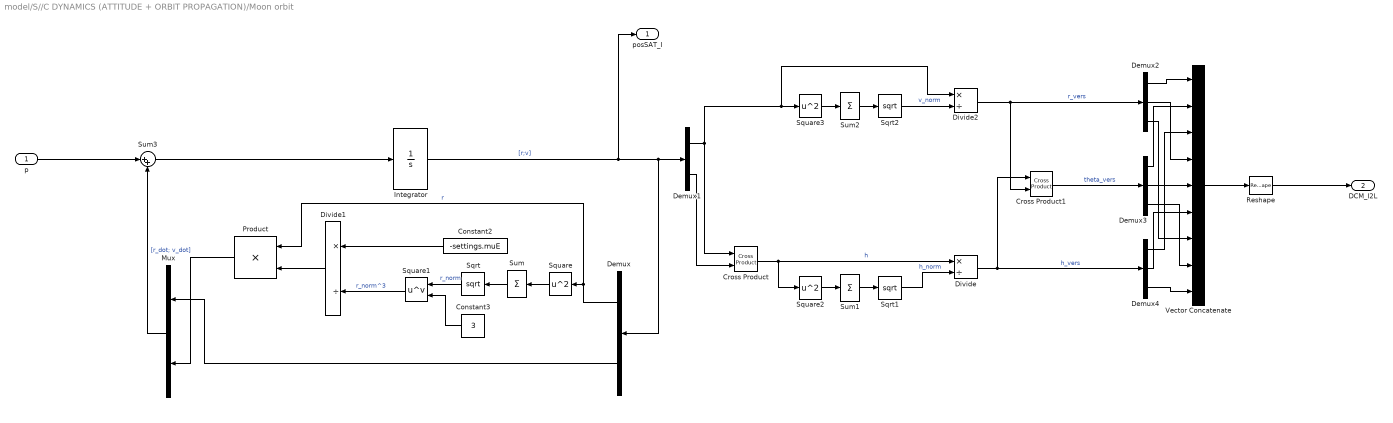
== system model/S//C DYNAMICS (ATTITUDE + ORBIT PROPAGATION)/Moon orbit ==
  p : Inport
  Constant2 : Constant  Value=-settings.muE
  Constant3 : Constant  Value=3
  Cross Product : vrlib/Utilities/Cross Product
  Cross Product1 : vrlib/Utilities/Cross Product
  Demux : Demux  Outputs=2
  Demux1 : Demux  Outputs=2
  Demux2 : Demux  Outputs=3
  Demux3 : Demux  Outputs=3
  Demux4 : Demux  Outputs=3
  Divide : Product  Inputs=*/
  Divide1 : Product  Inputs=*/
  Divide2 : Product  Inputs=*/
  Integrator : Integrator  InitialCondition=settings.Y0
  Mux : Mux  Inputs=2
  Product : Product
  Reshape : Reshape  OutputDimensionality=Customize  OutputDimensions=[3,3]
  Sqrt : Sqrt  SaturateOnIntegerOverflow=on
  Sqrt1 : Sqrt  SaturateOnIntegerOverflow=on
  Sqrt2 : Sqrt  SaturateOnIntegerOverflow=on
  Square : Math  Operator=square  SaturateOnIntegerOverflow=on
  Square1 : Math  Operator=pow  SaturateOnIntegerOverflow=on
  Square2 : Math  Operator=square  SaturateOnIntegerOverflow=on
  Square3 : Math  Operator=square  SaturateOnIntegerOverflow=on
  Sum : Sum  Inputs=+
  Sum1 : Sum  Inputs=+
  Sum2 : Sum  Inputs=+
  Sum3 : Sum  Inputs=|++
  Vector Concatenate : Concatenate  NumInputs=9
  posSAT_I : Outport
  DCM_I2L : Outport  Port=2
  wires:
  Constant3/1 -> Square1/2
  Demux/1 -> Product/1, Square/1  "r"
  Demux/2 -> Mux/1
  Integrator/1 -> Demux1/1, Demux/1, posSAT_I/1  "[r;v]"
  Divide1/1 -> Product/2
  Sqrt/1 -> Square1/1  "r_norm"
  Constant2/1 -> Divide1/1
  Product/1 -> Mux/2
  Sum/1 -> Sqrt/1
  Square/1 -> Sum/1
  Square1/1 -> Divide1/2  "r_norm^3"
  Mux/1 -> Sum3/2  "[r_dot; v_dot]"
  Sqrt2/1 -> Divide2/2  "v_norm"
  Divide2/1 -> Cross Product1/2, Demux2/1  "r_vers"
  Demux1/1 -> Cross Product/1, Divide2/1, Square3/1
  Demux2/2 -> Vector Concatenate/4
  Sqrt1/1 -> Divide/2  "h_norm"
  Demux4/1 -> Vector Concatenate/3
  Demux4/3 -> Vector Concatenate/9
  Demux3/3 -> Vector Concatenate/8
  Demux4/2 -> Vector Concatenate/6
  Vector Concatenate/1 -> Reshape/1
  Divide/1 -> Cross Product1/1, Demux4/1  "h_vers"
  Demux3/1 -> Vector Concatenate/2
  Sum1/1 -> Sqrt1/1
  Demux2/3 -> Vector Concatenate/7
  Square2/1 -> Sum1/1
  Demux2/1 -> Vector Concatenate/1
  Demux3/2 -> Vector Concatenate/5
  Cross Product/1 -> Divide/1, Square2/1  "h"
  Square3/1 -> Sum2/1
  Sum2/1 -> Sqrt2/1
  Cross Product1/1 -> Demux3/1  "theta_vers"
  Reshape/1 -> DCM_I2L/1
  Demux1/2 -> Cross Product/2
  Sum3/1 -> Integrator/1
  p/1 -> Sum3/1

== system model/S//C DYNAMICS (ATTITUDE + ORBIT PROPAGATION)/Orbit perturbations ==
  "[r;v]" : Inport
  Constant : Constant  Value=settings.orbitPert.J2
  If : If  IfExpression=u1
  J2 perturbation : Subsystem
  Terminator : Terminator
  if J2 perturbation : Subsystem  TreatAsAtomicUnit=on
  p : Outport
  wires:
  "[r;v]"/1 -> if J2 perturbation/1("[r;v]1")
  if J2 perturbation/1(Out1) -> J2 perturbation/1("[r;v]")
  J2 perturbation/1(p) -> p/1
  Constant/1 -> If/1
  If/2 -> Terminator/1
  If/1 -> if J2 perturbation/Action

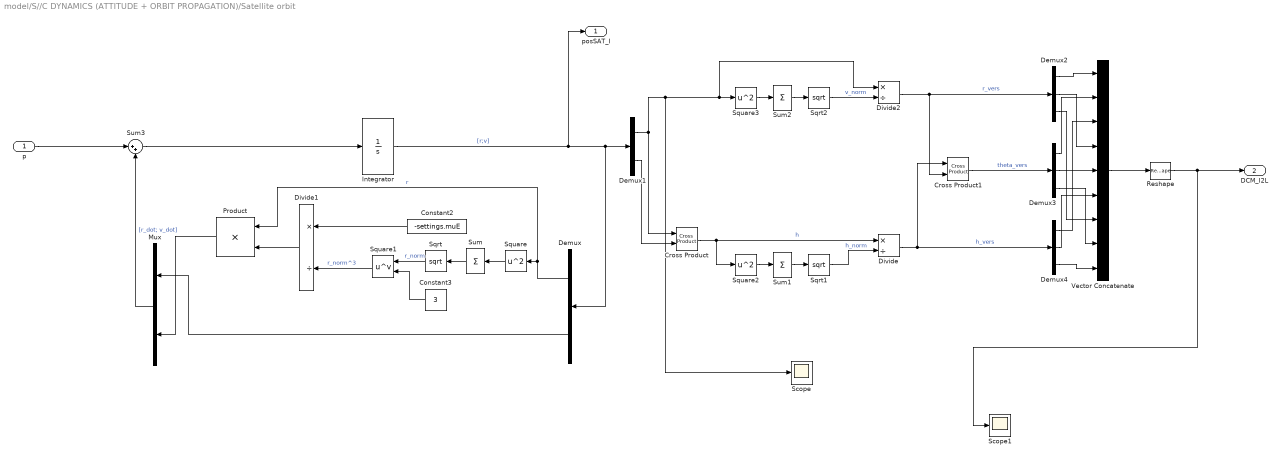
== system model/S//C DYNAMICS (ATTITUDE + ORBIT PROPAGATION)/Satellite orbit ==
  p : Inport
  Constant2 : Constant  Value=-settings.muE
  Constant3 : Constant  Value=3
  Cross Product : vrlib/Utilities/Cross Product
  Cross Product1 : vrlib/Utilities/Cross Product
  Demux : Demux  Outputs=2
  Demux1 : Demux  Outputs=2
  Demux2 : Demux  Outputs=3
  Demux3 : Demux  Outputs=3
  Demux4 : Demux  Outputs=3
  Divide : Product  Inputs=*/
  Divide1 : Product  Inputs=*/
  Divide2 : Product  Inputs=*/
  Integrator : Integrator  InitialCondition=settings.Y0
  Mux : Mux  Inputs=2
  Product : Product
  Reshape : Reshape  OutputDimensionality=Customize  OutputDimensions=[3,3]
  Scope : Scope
  Scope1 : Scope
  Sqrt : Sqrt  SaturateOnIntegerOverflow=on
  Sqrt1 : Sqrt  SaturateOnIntegerOverflow=on
  Sqrt2 : Sqrt  SaturateOnIntegerOverflow=on
  Square : Math  Operator=square  SaturateOnIntegerOverflow=on
  Square1 : Math  Operator=pow  SaturateOnIntegerOverflow=on
  Square2 : Math  Operator=square  SaturateOnIntegerOverflow=on
  Square3 : Math  Operator=square  SaturateOnIntegerOverflow=on
  Sum : Sum  Inputs=+
  Sum1 : Sum  Inputs=+
  Sum2 : Sum  Inputs=+
  Sum3 : Sum  Inputs=|++
  Vector Concatenate : Concatenate  NumInputs=9
  posSAT_I : Outport
  DCM_I2L : Outport  Port=2
  wires:
  Constant3/1 -> Square1/2
  Demux/1 -> Product/1, Square/1  "r"
  Demux/2 -> Mux/1
  Integrator/1 -> Demux1/1, Demux/1, posSAT_I/1  "[r;v]"
  Divide1/1 -> Product/2
  Sqrt/1 -> Square1/1  "r_norm"
  Constant2/1 -> Divide1/1
  Product/1 -> Mux/2
  Sum/1 -> Sqrt/1
  Square/1 -> Sum/1
  Square1/1 -> Divide1/2  "r_norm^3"
  Mux/1 -> Sum3/2  "[r_dot; v_dot]"
  Sqrt2/1 -> Divide2/2  "v_norm"
  Divide2/1 -> Cross Product1/2, Demux2/1  "r_vers"
  Demux1/1 -> Cross Product/1, Scope/1, Divide2/1, Square3/1
  Demux2/2 -> Vector Concatenate/4
  Sqrt1/1 -> Divide/2  "h_norm"
  Demux4/1 -> Vector Concatenate/3
  Demux4/3 -> Vector Concatenate/9
  Demux3/3 -> Vector Concatenate/8
  Demux4/2 -> Vector Concatenate/6
  Vector Concatenate/1 -> Reshape/1
  Divide/1 -> Cross Product1/1, Demux4/1  "h_vers"
  Demux3/1 -> Vector Concatenate/2
  Sum1/1 -> Sqrt1/1
  Demux2/3 -> Vector Concatenate/7
  Square2/1 -> Sum1/1
  Demux2/1 -> Vector Concatenate/1
  Demux3/2 -> Vector Concatenate/5
  Cross Product/1 -> Divide/1, Square2/1  "h"
  Square3/1 -> Sum2/1
  Sum2/1 -> Sqrt2/1
  Cross Product1/1 -> Demux3/1  "theta_vers"
  Reshape/1 -> Scope1/1, DCM_I2L/1
  Demux1/2 -> Cross Product/2
  Sum3/1 -> Integrator/1
  p/1 -> Sum3/1

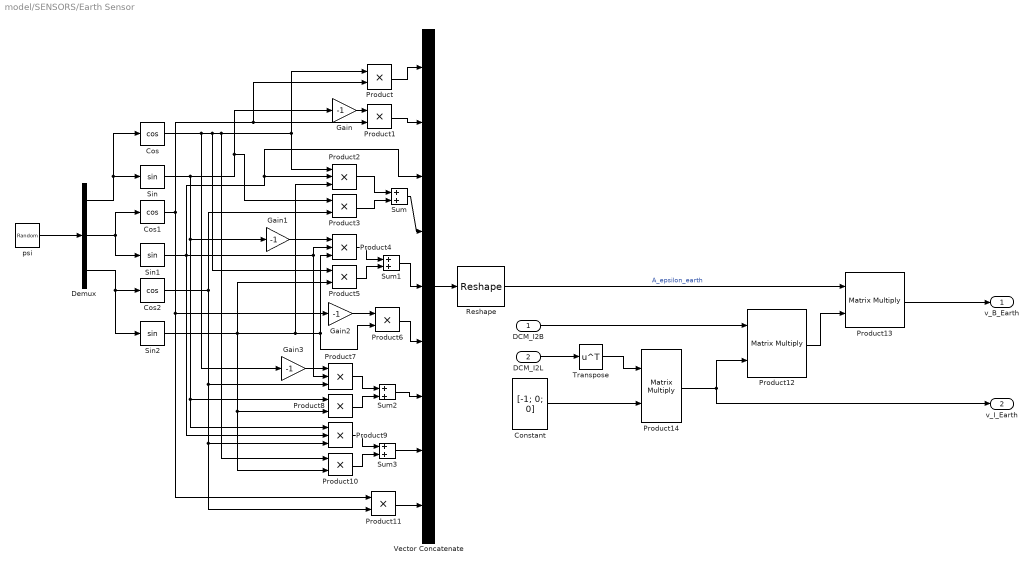
== system model/SENSORS/Earth Sensor ==
  DCM_I2B : Inport
  DCM_I2L : Inport  Port=2
  Constant : Constant  Value=[-1; 0; 0]
  Cos : Trigonometry  Operator=cos
  Cos1 : Trigonometry  Operator=cos
  Cos2 : Trigonometry  Operator=cos
  Demux : Demux  Outputs=3
  Gain{,1..3} (4 alike) : Gain  Gain=-1
  Product{,1,3,5..6,8,10..11} (8 alike) : Product
  Product12 : Product  Multiplication=Matrix(*)
  Product13 : Product  Multiplication=Matrix(*)
  Product14 : Product  Multiplication=Matrix(*)
  Product{2,4,7,9} (4 alike) : Product  Inputs=3
  Reshape : Reshape  OutputDimensionality=Customize  OutputDimensions=[3,3]
  Sin : Trigonometry
  Sin1 : Trigonometry
  Sin2 : Trigonometry
  Sum{,1..3} (4 alike) : Sum
  Transpose : Math  Operator=transpose  SaturateOnIntegerOverflow=on
  Vector Concatenate : Concatenate  NumInputs=9
  psi : RandomNumber  Variance=(1/4 * deg2rad(settings.EarthSensorAccuracy * [1 1 1])).^2  Seed=[4 5 6]  SampleTime=0.1
  v_B_Earth : Outport
  v_I_Earth : Outport  Port=2
  wires:
  Cos/1 -> Gain3/1, Product5/1, Product10/1, Product2/1, Product/1
  Cos1/1 -> Product11/1, Gain2/1, Product1/2, Product/2
  Product/1 -> Vector Concatenate/1
  Product1/1 -> Vector Concatenate/2
  Gain/1 -> Product1/1
  Sin/1 -> Product9/1, Product8/1, Gain1/1, Product3/1, Gain/1
  Sin1/1 -> Product9/2, Product7/2, Product4/2, Product2/2, Vector Concatenate/3
  Sin2/1 -> Product10/2, Product8/2, Product6/2, Product4/3, Product2/3, Product5/2
  Sum/1 -> Vector Concatenate/4
  Product2/1 -> Sum/1
  Product3/1 -> Sum/2
  Cos2/1 -> Product11/2, Product9/3, Product7/3, Product3/2
  Product5/1 -> Sum1/2
  Product4/1 -> Sum1/1
  Sum1/1 -> Vector Concatenate/5
  Gain1/1 -> Product4/1
  Product6/1 -> Vector Concatenate/6
  Gain2/1 -> Product6/1
  Product7/1 -> Sum2/1
  Product8/1 -> Sum2/2
  Sum2/1 -> Vector Concatenate/7
  Gain3/1 -> Product7/1
  Product10/1 -> Sum3/2
  Product9/1 -> Sum3/1
  Sum3/1 -> Vector Concatenate/8
  Product11/1 -> Vector Concatenate/9
  Vector Concatenate/1 -> Reshape/1
  Reshape/1 -> Product13/1  "A_epsilon_earth"
  DCM_I2B/1 -> Product12/1
  Product12/1 -> Product13/2
  Product13/1 -> v_B_Earth/1
  Product14/1 -> Product12/2, v_I_Earth/1
  Constant/1 -> Product14/2
  DCM_I2L/1 -> Transpose/1
  Demux/2 -> Sin1/1, Cos1/1
  Demux/3 -> Cos2/1, Sin2/1
  Demux/1 -> Cos/1, Sin/1
  psi/1 -> Demux/1
  Transpose/1 -> Product14/1

== system model/SENSORS/Gyroscope ==
  omega : Inport
  ARW : RandomNumber  Variance=(1/4*deg2rad(settings.GyroscopeARW*[1;1;1]/sqrt(3600))).^2  Seed=1  SampleTime=1/settings.GyroscopeSampleRate
  Integrator : Integrator
  Integrator1 : Integrator  InitialCondition=[0 0 0 0 0 0]'
  MATLAB Function : MATLAB Function  TreatAsAtomicUnit=on
  MATLAB Function1 : MATLAB Function  TreatAsAtomicUnit=on
  RRW : RandomNumber  Variance=(1/4*deg2rad(settings.GyroscopeRRW*[1;1;1]/3600^3)).^2  Seed=2  SampleTime=1/settings.GyroscopeSampleRate
  Sum : Sum  Inputs=+++
  omega_sens : Outport
  wires:
  Sum/1 -> MATLAB Function/2(om)
  RRW/1 -> Integrator/1
  ARW/1 -> Sum/2
  Integrator/1 -> Sum/3
  omega/1 -> Sum/1
  MATLAB Function/1(x_dot) -> Integrator1/1
  Integrator1/1 -> MATLAB Function1/1(state_vector), MATLAB Function/1(x)
  MATLAB Function1/1(omega_raw) -> omega_sens/1

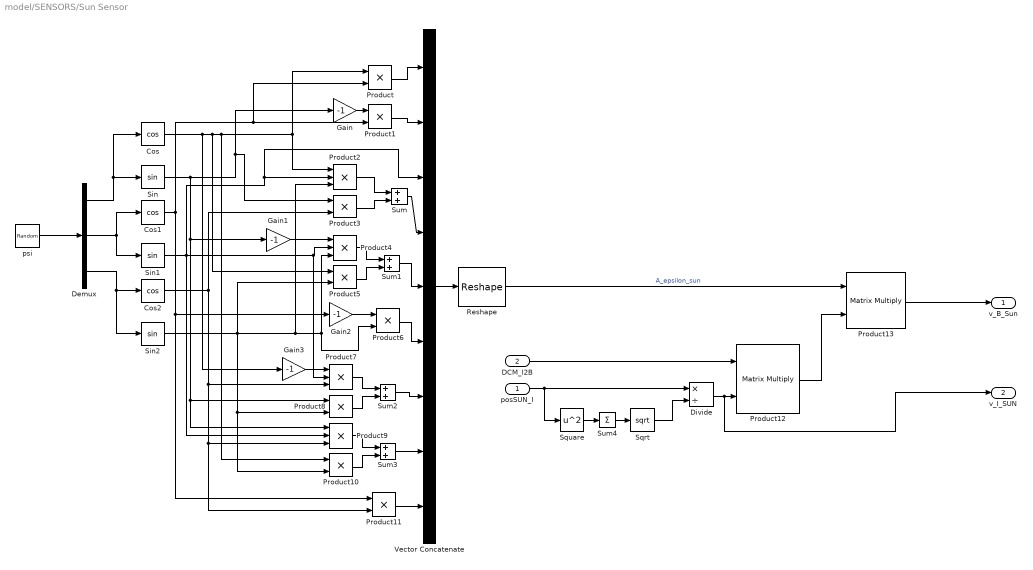
== system model/SENSORS/Sun Sensor ==
  posSUN_I : Inport
  DCM_I2B : Inport  Port=2
  Cos : Trigonometry  Operator=cos
  Cos1 : Trigonometry  Operator=cos
  Cos2 : Trigonometry  Operator=cos
  Demux : Demux  Outputs=3
  Divide : Product  Inputs=*/
  Gain{,1..3} (4 alike) : Gain  Gain=-1
  Product{,1,3,5..6,8,10..11} (8 alike) : Product
  Product12 : Product  Multiplication=Matrix(*)
  Product13 : Product  Multiplication=Matrix(*)
  Product{2,4,7,9} (4 alike) : Product  Inputs=3
  Reshape : Reshape  OutputDimensionality=Customize  OutputDimensions=[3,3]
  Sin : Trigonometry
  Sin1 : Trigonometry
  Sin2 : Trigonometry
  Sqrt : Sqrt  SaturateOnIntegerOverflow=on
  Square : Math  Operator=square  SaturateOnIntegerOverflow=on
  Sum{,1..3} (4 alike) : Sum
  Sum4 : Sum  Inputs=+
  Vector Concatenate : Concatenate  NumInputs=9
  psi : RandomNumber  Variance=(1/4 * deg2rad(settings.SunSensorAccuracy * [1 1 1])).^2  Seed=[1 2 3]  SampleTime=0.1
  v_B_Sun : Outport
  v_I_SUN : Outport  Port=2
  wires:
  Demux/2 -> Sin1/1, Cos1/1
  Demux/3 -> Sin2/1, Cos2/1
  Cos/1 -> Gain3/1, Product5/1, Product10/1, Product2/1, Product/1
  Cos1/1 -> Product11/1, Gain2/1, Product1/2, Product/2
  Product/1 -> Vector Concatenate/1
  Product1/1 -> Vector Concatenate/2
  Gain/1 -> Product1/1
  Sin/1 -> Product9/1, Product8/1, Gain1/1, Product3/1, Gain/1
  Sin1/1 -> Product9/2, Product7/2, Product4/2, Product2/2, Vector Concatenate/3
  Sin2/1 -> Product10/2, Product8/2, Product6/2, Product4/3, Product2/3, Product5/2
  Sum/1 -> Vector Concatenate/4
  Product2/1 -> Sum/1
  Product3/1 -> Sum/2
  Cos2/1 -> Product11/2, Product9/3, Product7/3, Product3/2
  Product5/1 -> Sum1/2
  Product4/1 -> Sum1/1
  Sum1/1 -> Vector Concatenate/5
  Gain1/1 -> Product4/1
  Product6/1 -> Vector Concatenate/6
  Gain2/1 -> Product6/1
  Product7/1 -> Sum2/1
  Product8/1 -> Sum2/2
  Sum2/1 -> Vector Concatenate/7
  Gain3/1 -> Product7/1
  Product10/1 -> Sum3/2
  Product9/1 -> Sum3/1
  Sum3/1 -> Vector Concatenate/8
  Product11/1 -> Vector Concatenate/9
  Vector Concatenate/1 -> Reshape/1
  Reshape/1 -> Product13/1  "A_epsilon_sun"
  DCM_I2B/1 -> Product12/1
  posSUN_I/1 -> Divide/1, Square/1
  Square/1 -> Sum4/1
  Sum4/1 -> Sqrt/1
  Product12/1 -> Product13/2
  Product13/1 -> v_B_Sun/1
  Demux/1 -> Sin/1, Cos/1
  psi/1 -> Demux/1
  Divide/1 -> v_I_SUN/1, Product12/2
  Sqrt/1 -> Divide/2

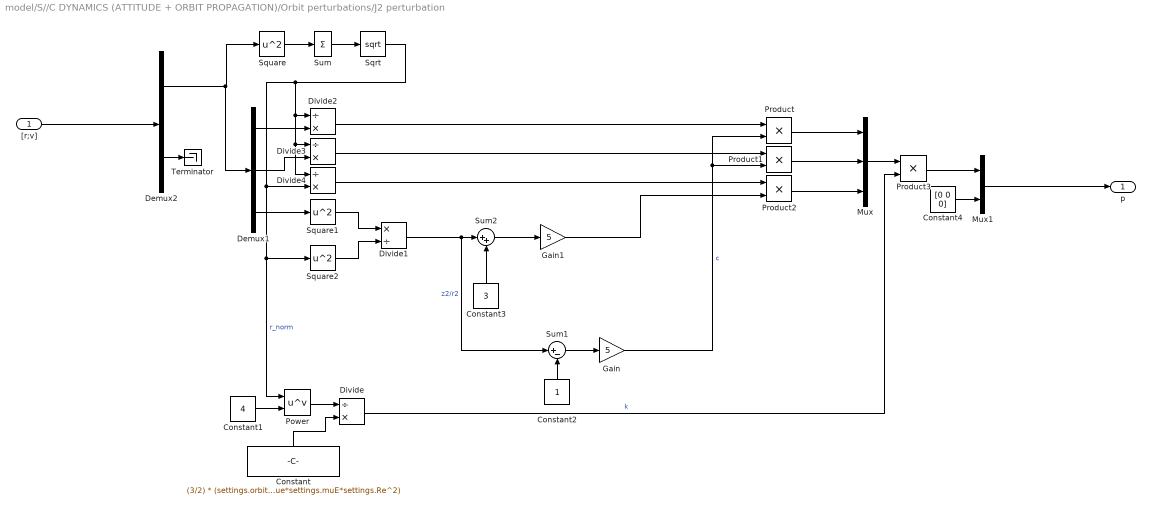
== system model/S//C DYNAMICS (ATTITUDE + ORBIT PROPAGATION)/Orbit perturbations/J2 perturbation ==
  "[r;v]" : Inport
  Constant : Constant  Value=(3/2) * (settings.orbitPert.J2value*settings.muE*settings.Re^2)
  Constant1 : Constant  Value=4
  Constant2 : Constant
  Constant3 : Constant  Value=3
  Constant4 : Constant  Value=[0 0 0]
  Demux1 : Demux  Outputs=3
  Demux2 : Demux  Outputs=2
  Divide{,2..4} (4 alike) : Product  Inputs=/*
  Divide1 : Product  Inputs=*/
  Gain : Gain  Gain=5
  Gain1 : Gain  Gain=5
  Mux : Mux  Inputs=3
  Mux1 : Mux  Inputs=2
  Power : Math  Operator=pow  SaturateOnIntegerOverflow=on
  Product{,1..3} (4 alike) : Product
  Sqrt : Sqrt  SaturateOnIntegerOverflow=on
  Square : Math  Operator=square  SaturateOnIntegerOverflow=on
  Square1 : Math  Operator=square  SaturateOnIntegerOverflow=on
  Square2 : Math  Operator=square  SaturateOnIntegerOverflow=on
  Sum : Sum  Inputs=+
  Sum1 : Sum  Inputs=|+-
  Sum2 : Sum  Inputs=|++
  Terminator : Terminator
  p : Outport
  wires:
  "[r;v]"/1 -> Demux2/1
  Demux2/2 -> Terminator/1
  Square/1 -> Sum/1
  Sum/1 -> Sqrt/1
  Sqrt/1 -> Divide4/1, Divide3/1, Divide2/1, Divide4/2, Power/1, Square2/1  "r_norm"
  Demux2/1 -> Demux1/1, Square/1
  Constant/1 -> Divide/2
  Constant1/1 -> Power/2
  Power/1 -> Divide/1
  Demux1/3 -> Square1/1
  Square1/1 -> Divide1/1
  Square2/1 -> Divide1/2
  Constant2/1 -> Sum1/2
  Divide1/1 -> Sum1/1, Sum2/1  "z2/r2"
  Sum1/1 -> Gain/1
  Gain/1 -> Product1/2, Product/2  "c"
  Divide/1 -> Product3/2  "k"
  Demux1/1 -> Divide2/2
  Divide2/1 -> Product/1
  Demux1/2 -> Divide3/2
  Divide3/1 -> Product1/1
  Constant3/1 -> Sum2/2
  Sum2/1 -> Gain1/1
  Divide4/1 -> Product2/1
  Gain1/1 -> Product2/2
  Product/1 -> Mux/1
  Product1/1 -> Mux/2
  Product2/1 -> Mux/3
  Mux/1 -> Product3/1
  Product3/1 -> Mux1/1
  Constant4/1 -> Mux1/2
  Mux1/1 -> p/1

== system model/S//C DYNAMICS (ATTITUDE + ORBIT PROPAGATION)/Orbit perturbations/if J2 perturbation ==
  "[r;v]1" : Inport
  Action Port : ActionPort  ActionPortLabel=if(u1)
  Out1 : Outport
  wires:
  "[r;v]1"/1 -> Out1/1

== matlab function model/CONTROL AND ACTUATORS/If Action Subsystem2/fcn ==
  data: A_BI_sensed input; S_I input; A_LI input; rv input; A_BI input; A_e output; w_req output; pointing_err output
function [A_e, w_req, pointing_err]  = fcn(A_BI_sensed, S_I, A_LI, rv, A_BI)
r = rv(1:3,1);
v = rv(4:6,1);

%% Calculating Target Attitude Matrix
X_B  = A_LI'*[-1;0;0];    % Inertial position of Earth
h_vers = cross(r,v)/norm(cross(r,v));
r_vers = r/norm(r);
trasversal_velocity_vers = cross(h_vers, r_vers);
Y_B = -trasversal_velocity_vers;
Z_B = cross(X_B,Y_B);

A_T = [X_B';Y_B';Z_B'];
A_e = A_BI_sensed*A_T';

%% Pointing Accuracy
X_B_actual = A_BI'*[1;0;0];
if abs(dot(X_B,X_B_actual)) > 1
    pointing_err = 0;
else
    pointing_err = rad2deg(acos(dot(X_B,X_B_actual)));
end

%% Calculating Target Angular Velocity
w_target = cross(r,v)/(norm(r)^2);

w_req = A_BI_sensed*A_LI'*w_target;

== matlab function model/CONTROL AND ACTUATORS/If Action Subsystem3/MATLAB Function ==
  data: rv input; w_e output; A_BI_sensed input; A_LI input; estW input; A_e output; A_BI input; pointing_err output
function [w_e, A_e, pointing_err]  = fcn(rv, A_BI_sensed, A_LI, estW, A_BI)
r = rv(1:3,1);
v = rv(4:6,1);

%% Calculating Target Attitude Matrix
X_B  = A_LI'*[-1;0;0];    % Inertial position of Earth
h_vers = cross(r,v)/norm(cross(r,v));
r_vers = r/norm(r);
trasversal_velocity_vers = cross(h_vers, r_vers);
Y_B = -trasversal_velocity_vers;
Z_B = cross(X_B,Y_B);

A_T = [X_B';Y_B';Z_B'];
A_e = A_BI_sensed*A_T';

w_target = cross(r,v)/(norm(r)^2);

w_e = estW - A_e*w_target;

X_B_actual = A_BI'*[1;0;0];
pointing_err = rad2deg(acos(dot(X_B,X_B_actual)));

== matlab function model/CONTROL AND ACTUATORS/If Action Subsystem3/MATLAB Function1 ==
  data: w_e input; Mc output; A_e input; estW input; estMD input; k1 input; k2 input; J input
function Mc = fcn(w_e, A_e, estW, estMD, k1, k2, J)

AeT_AeV = [A_e(2,3) - A_e(3,2), A_e(3,1) - A_e(1,3), A_e(1,2) - A_e(2,1)]';

Mc = -k1*w_e - k2*AeT_AeV + cross(estW, J*estW) - estMD;

== matlab function model/CONTROL AND ACTUATORS/Actual Torque produced by RW1 ==
  data: dwr input; MeffRW output; wr input; w input; Irw input
function MeffRW = fcn(dwr,wr,w,Irw)

A=[1 0 0; 0 1 0; 0 0 1];
Irw=Irw*eye(3);
hr=Irw*wr;
dhr=Irw*dwr;
MeffRW=-A*dhr-cross(w,A*hr);

== matlab function model/CONTROL AND ACTUATORS/MATLAB Function3 ==
  data: Mc input; w_b_sensed input; dwr output; Irw input; wr input
function dwr = fcn(Mc,w_b_sensed,Irw,wr)

A=[1 0 0; 0 1 0; 0 0 1];

Irwmat = Irw*eye(3);
hr = Irwmat*wr;
F = cross(A*hr,w_b_sensed)-Mc;
G = A\F;
dhr = G(1:3,1);
dwr = dhr/Irw;

== matlab function model/CONTROL AND ACTUATORS/fcn ==
  data: A_BI_sensed input; S_I input; A_LI input; rv input; A_BI input; A_e output; w_req output; pointing_err output
function [A_e, w_req, pointing_err]  = fcn(A_BI_sensed, S_I, A_LI, rv, A_BI)

%% Calculating Target Attitude Matrix
Z_B  = A_LI'*[-1;0;0];
sun_direction = S_I/norm(S_I);
X_B = sun_direction - dot(sun_direction,Z_B)*Z_B;
Y_B = cross(Z_B,X_B);

A_T = [X_B';Y_B';Z_B'];
A_e = A_BI_sensed*A_T';

%% Pointing Accuracy
Z_B_actual = A_BI'*[0;0;1];
pointing_err = rad2deg(acos(dot(Z_B,Z_B_actual)));

%% Calculating Target Angular Velocity
r = rv(1:3,1);
v = rv(4:6,1);

w_target = cross(r,v)/(norm(r)^2);

w_req = A_BI_sensed*A_LI'*w_target;

== matlab function model/CONTROL AND ACTUATORS/MATLAB Function ==
  data: MagMax input; B_sensed input; Mc input; D output; M_eff_sensed output
function [D, M_eff_sensed] = fcn(MagMax,B_sensed,Mc)
D=1/dot(B_sensed,B_sensed)*cross(B_sensed,Mc);
if D(1)>MagMax
    D(1)=MagMax;
end
if D(2)>MagMax
    D(2)=MagMax;
end
if D(3)>MagMax
    D(3)=MagMax;
end
M_eff_sensed=cross(D,B_sensed);

== matlab function model/CONTROL AND ACTUATORS/Actual Torque produced by RW ==
  data: dwr input; MeffRW output; wr input; w input; Irw input
function MeffRW = fcn(dwr,wr,w,Irw)

A=[1 0 0; 0 1 0; 0 0 1];
Irw=Irw*eye(3);
hr=Irw*wr;
dhr=Irw*dwr;
MeffRW=-A*dhr-cross(w,A*hr);

== matlab function model/CONTROL AND ACTUATORS/MATLAB Function1 ==
  data: Mc input; w_b_sensed input; dwr output; Irw input; wr input
function dwr = fcn(Mc,w_b_sensed,Irw,wr)

A=[1 0 0; 0 1 0; 0 0 1];

Irwmat = Irw*eye(3);
hr = Irwmat*wr;
F = cross(A*hr,w_b_sensed)-Mc;
G = A\F;
dhr = G(1:3,1);
dwr = dhr/Irw;

== matlab function model/CONTROL AND ACTUATORS/Target Pointing Algorithm ==
  data: w_b_sensed input; A_e input; Mc output; w_req input; Kp input; Kd input
function Mc  = fcn(w_b_sensed,A_e,w_req,Kp,Kd)

Mx = -Kp(1,1)/2*(A_e(2,3)-A_e(3,2))-Kd(1,1)*(w_b_sensed(1)-w_req(1));
My = -Kp(2,1)/2*(A_e(3,1)-A_e(1,3))-Kd(2,1)*(w_b_sensed(2)-w_req(2));
Mz = -Kp(3,1)/2*(A_e(1,2)-A_e(2,1))-Kd(3,1)*(w_b_sensed(3)-w_req(3));

Mc=[Mx;My;Mz];

== matlab function model/CONTROL AND ACTUATORS/RW Moment ==
  data: M_onlyMagnetorquer input; M_req_Detumbling input; RW_Moment output; M_Target_Pointing input; tMaxOnlyMagn input; tMaxDetumbling input; t input
function RW_Moment = fcn(M_onlyMagnetorquer, M_req_Detumbling, M_Target_Pointing, tMaxOnlyMagn, tMaxDetumbling, t)

if t <= tMaxOnlyMagn
    RW_Moment = [0 0 0]';
elseif t > tMaxOnlyMagn && t <= tMaxDetumbling
    RW_Moment = M_req_Detumbling;
else
    RW_Moment = M_Target_Pointing;
end

== matlab function model/SENSORS/SVD ==
  data: B input; A_BI_sensed output
function A_BI_sensed = fcn(B)

[U, ~, V] = svd(B);
M = diag([1, 1, det(U)* det(V)]);
A_BI_sensed = U*M*V';

end
